simulink model "Driveline_ctrl_sim_Int"  (R2020a)
settings: Solver=VariableStepAuto  StartTime=0.0  StopTime=50  RelTol=1e-3
values from neighbouring files (symbols this model uses):
  A = [[-1/tau 0];[1/m -rho*CD*Af*x2e/m]]    [CruiseCtrl_StateFeedback_Int_design.m]
  B = [k*r/tau/rw 0]'    [CruiseCtrl_StateFeedback_Int_design.m]
  C = [0 1]    [CruiseCtrl_StateFeedback_Int_design.m]
  D = [0]    [CruiseCtrl_StateFeedback_Int_design.m]
undefined symbols (not defined in the file or in its folder): G, K, ki, kr, M, phi, R, x0
libraries: simulink_extras x1
settings Model: Creator=juan  LastModifiedBy=juan

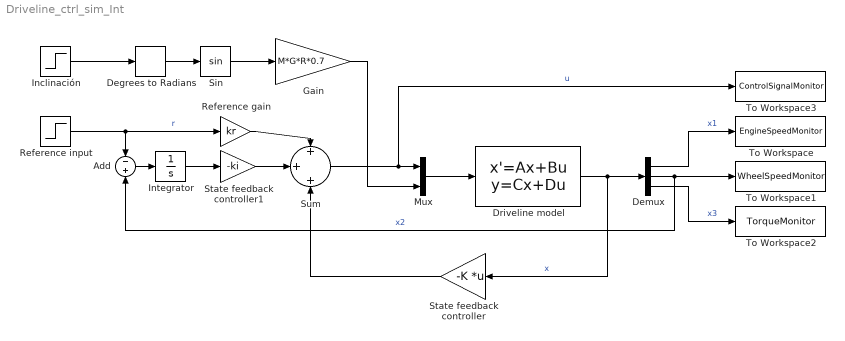
== system Driveline_ctrl_sim_Int ==
  Add : Sum  Inputs=-+
  Degrees to Radians : simulink_extras/Transformations/Degrees to Radians
  Demux : Demux  Outputs=3
  Driveline model : StateSpace  A=A  B=B  C=C  D=D  InitialCondition=x0
  Gain : Gain  Gain=M*G*R*0.7
  Inclinación : Step  Time=10  After=phi  SampleTime=0
  Integrator : Integrator
  Mux : Mux  Inputs=2
  Reference gain : Gain  Gain=kr
  Reference input : Step  Before=2  After=4  SampleTime=0
  Sin : Trigonometry
  State feedback controller : Gain  Gain=-K  Multiplication=Matrix(K*u)
  State feedback controller1 : Gain  Gain=-ki
  Sum : Sum  Inputs=+|+|+
  To Workspace : ToWorkspace  VariableName=EngineSpeedMonitor  SaveFormat=Structure With Time  SampleTime=-1
  To Workspace1 : ToWorkspace  VariableName=WheelSpeedMonitor  SaveFormat=Structure With Time  SampleTime=-1
  To Workspace2 : ToWorkspace  VariableName=TorqueMonitor  SaveFormat=Structure With Time  SampleTime=-1
  To Workspace3 : ToWorkspace  VariableName=ControlSignalMonitor  SaveFormat=Structure With Time  SampleTime=-1
  wires:
  Sin/1 -> Gain/1
  Degrees to Radians/1 -> Sin/1
  Demux/2 -> To Workspace1/1, Add/2  "x2"
  Demux/3 -> To Workspace2/1  "x3"
  Inclinación/1 -> Degrees to Radians/1
  Reference gain/1 -> Sum/1
  Sum/1 -> To Workspace3/1, Mux/1  "u"
  Demux/1 -> To Workspace/1  "x1"
  Gain/1 -> Mux/2
  Mux/1 -> Driveline model/1
  Reference input/1 -> Reference gain/1, Add/1  "r"
  Driveline model/1 -> Demux/1, State feedback controller/1  "x"
  State feedback controller/1 -> Sum/3
  Add/1 -> Integrator/1
  State feedback controller1/1 -> Sum/2
  Integrator/1 -> State feedback controller1/1
